simulink model "VelocityControlPI"  (R2022a)
settings: Solver=VariableStepAuto  StartTime=0.0  StopTime=inf  RelTol=1e-3
undefined symbols (not defined in the file): a, b, k1, k2
libraries: arduinolib x4, arduinosensorlib x2
settings Model: Creator=LabPC  LastModifiedBy=LabPC

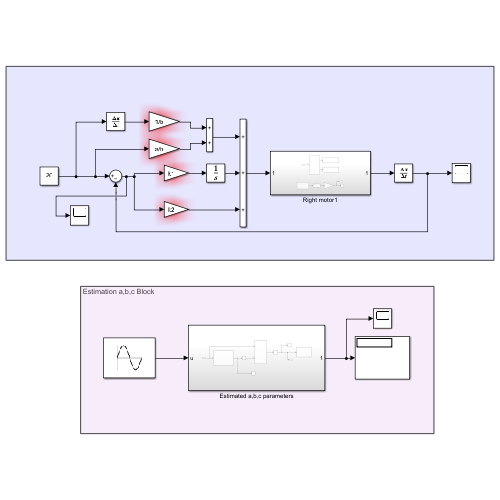
[thumbnail: Simulink's stored preview of the top-level diagram]
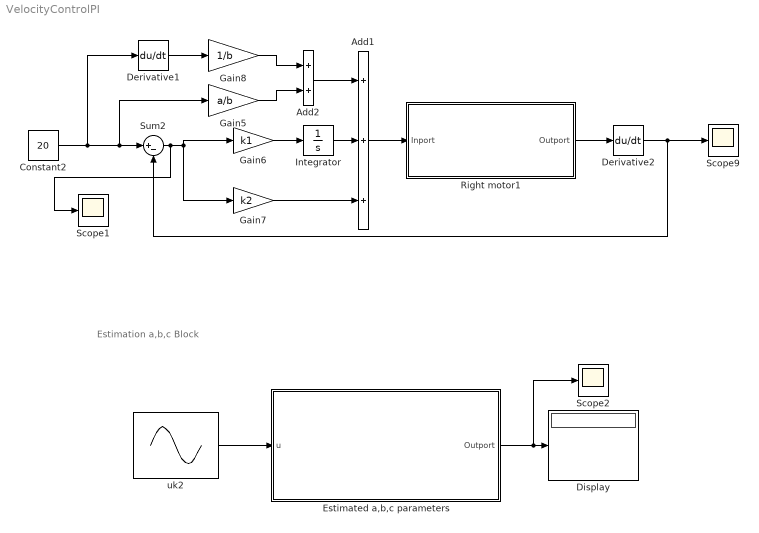
== system VelocityControlPI ==
  note: Estimation a,b,c Block
  Add1 : Sum  Inputs=+++
  Add2 : Sum
  Constant2 : Constant  Value=20
  Derivative1 : Derivative
  Derivative2 : Derivative
  Display : Display
  Estimated a,b,c parameters : Subsystem
  Gain5 : Gain  Gain=a/b
  Gain6 : Gain  Gain=k1
  Gain7 : Gain  Gain=k2
  Gain8 : Gain  Gain=1/b
  Integrator : Integrator
  Right motor1 : Subsystem
  Scope1 : Scope
  Scope2 : Scope
  Scope9 : Scope
  Sum2 : Sum  Inputs=|+-
  uk2 : Sin  Amplitude=14  Frequency=2*pi*1  SampleTime=0
  wires:
  Gain8/1 -> Add2/1
  Gain6/1 -> Integrator/1
  Right motor1/1(Outport) -> Derivative2/1
  Sum2/1 -> Scope1/1, Gain6/1, Gain7/1
  Derivative1/1 -> Gain8/1
  Integrator/1 -> Add1/2
  Add1/1 -> Right motor1/1(Inport)
  Add2/1 -> Add1/1
  Derivative2/1 -> Scope9/1, Sum2/2
  Gain7/1 -> Add1/3
  Gain5/1 -> Add2/2
  Constant2/1 -> Gain5/1, Sum2/1, Derivative1/1
  uk2/1 -> Estimated a,b,c parameters/1(u)
  Estimated a,b,c parameters/1(Outport) -> Scope2/1, Display/1

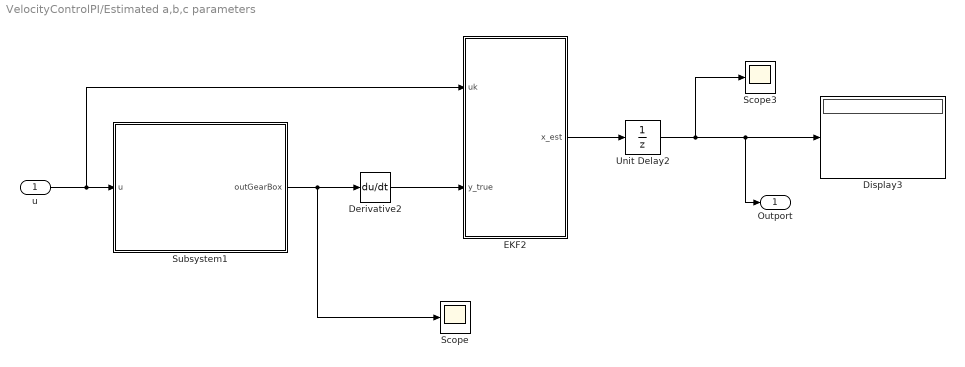
== system VelocityControlPI/Estimated a,b,c parameters ==
  u : Inport
  Derivative2 : Derivative
  Display3 : Display
  EKF2 : MATLAB Function  TreatAsAtomicUnit=on
  Scope : Scope
  Scope3 : Scope
  Subsystem1 : Subsystem
  Unit Delay2 : UnitDelay  InitialCondition=[0;0;0;0]  SampleTime=-1  HasFrameUpgradeWarning=on
  Outport : Outport
  wires:
  Derivative2/1 -> EKF2/2(y_true)
  Unit Delay2/1 -> Outport/1, Display3/1, Scope3/1
  EKF2/1(x_est) -> Unit Delay2/1
  Subsystem1/1(outGearBox) -> Scope/1, Derivative2/1
  u/1 -> EKF2/1(uk), Subsystem1/1(u)

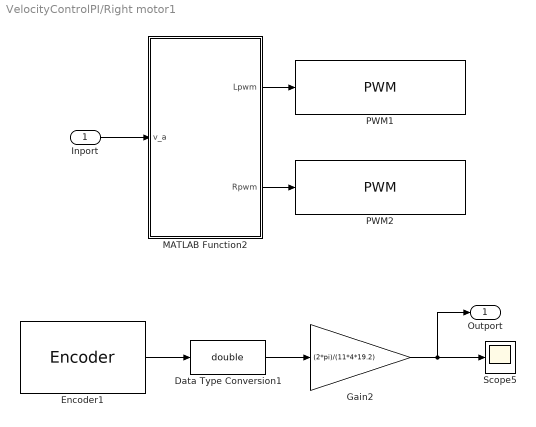
== system VelocityControlPI/Right motor1 ==
  Inport : Inport
  Data Type Conversion1 : DataTypeConversion  OutDataTypeStr=double  SaturateOnIntegerOverflow=off  RndMeth=Floor
  Encoder1 : arduinosensorlib/Encoder  InputA=2  InputB=3  Mode=No reset  SampleTime=-1
      settings: SourceProductBaseCode=ARDUINO
  Gain2 : Gain  Gain=(2*pi)/(11*4*19.2)
  MATLAB Function2 : MATLAB Function  TreatAsAtomicUnit=on
  PWM1 : arduinolib/PWM  pinNumber=8  frequencyType=Default  desiredFrequency=490.2  achievableFrequency=490.2
  PWM2 : arduinolib/PWM  pinNumber=9  frequencyType=Default  desiredFrequency=490.2  achievableFrequency=490.2
  Scope5 : Scope
  Outport : Outport
  wires:
  Gain2/1 -> Scope5/1, Outport/1
  Data Type Conversion1/1 -> Gain2/1
  Encoder1/1 -> Data Type Conversion1/1
  Inport/1 -> MATLAB Function2/1(v_a)
  MATLAB Function2/1(Lpwm) -> PWM1/1
  MATLAB Function2/2(Rpwm) -> PWM2/1

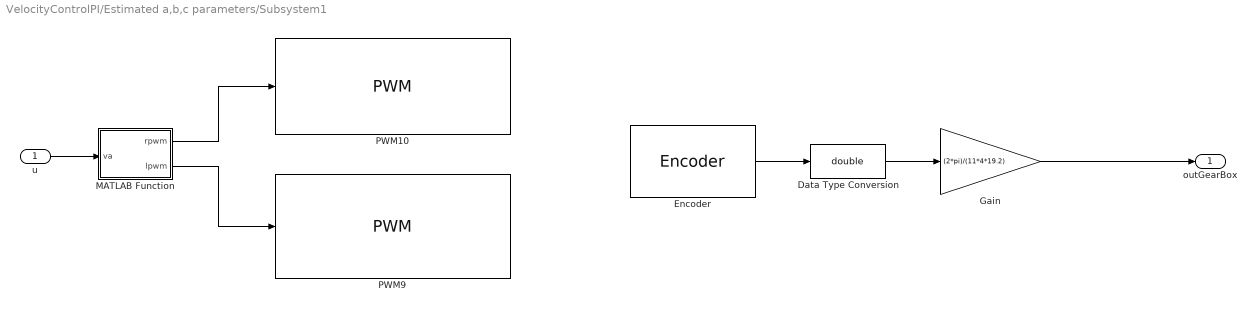
== system VelocityControlPI/Estimated a,b,c parameters/Subsystem1 ==
  u : Inport
  Data Type Conversion : DataTypeConversion  OutDataTypeStr=double  SaturateOnIntegerOverflow=off  RndMeth=Floor
  Encoder : arduinosensorlib/Encoder  InputA=2  InputB=3  Mode=No reset  SampleTime=-1
      settings: SourceProductBaseCode=ARDUINO
  Gain : Gain  Gain=(2*pi)/(11*4*19.2)
  MATLAB Function : MATLAB Function  TreatAsAtomicUnit=on
  PWM10 : arduinolib/PWM  pinNumber=8  frequencyType=Default  desiredFrequency=490.2  achievableFrequency=490.2
  PWM9 : arduinolib/PWM  pinNumber=9  frequencyType=Default  desiredFrequency=490.2  achievableFrequency=490.2
  outGearBox : Outport
  wires:
  Gain/1 -> outGearBox/1
  u/1 -> MATLAB Function/1(va)
  MATLAB Function/1(rpwm) -> PWM10/1
  MATLAB Function/2(lpwm) -> PWM9/1
  Encoder/1 -> Data Type Conversion/1
  Data Type Conversion/1 -> Gain/1

== matlab function VelocityControlPI/Estimated a,b,c parameters/Subsystem1/MATLAB Function ==
  data: va input; rpwm output; lpwm output
function [rpwm,lpwm] = fcn(va)

pwm = (va/24)*254;

if pwm > 0
    rpwm = pwm;
    lpwm = 0;
elseif pwm<0
    rpwm = 0;
    lpwm = abs(pwm);
else
    rpwm = 0;
    lpwm = 0;
end

== matlab function VelocityControlPI/Right motor1/MATLAB Function2 ==
  data: v_a input; Lpwm output; Rpwm output
function [Lpwm,Rpwm] = fcn(v_a)

vmax = 22.9;
pwm_cal = v_a*254/vmax;

if pwm_cal > 0
    Lpwm = 0;
    Rpwm = pwm_cal;
elseif pwm_cal < 0
    Lpwm = abs(pwm_cal);
    Rpwm = 0;
else
    Lpwm = 0;
    Rpwm = 0;
end

== matlab function VelocityControlPI/Estimated a,b,c parameters/EKF2 ==
  settings: updateMethod=DISCRETE
  data: uk input; y_true input; x_est output
function x_est = fcn(uk,y_true)
Ts=0.01;
persistent x_est_p P Qd_est R_est Qc_est;
if isempty(x_est_p)
          
          x_est_p=[2;13;25;1];
          P=2*eye(4);
         Qc_est=1e-5*diag([10,25,25,1]);
          Qd_est=Qc_est*Ts;
          R_est=0.02;
end
c=[1 0 0 0];D=0;Ck=c;Dk=D;
%Comput Kalman Gain and update predicted value
Wk=P*Ck'/(Ck*P*Ck'+R_est);
y_est=Ck*x_est_p+Dk*uk;
x=x_est_p+Wk.*(y_true-y_est);
%Compute prediction at next time step
x_est=x+Ts*[-x(2)*x(1)+uk*x(3)-x(4)*sign(x(1));0;0;0];
%Update error covariance matrices
P=P-Wk*Ck*P;
%Define Ak
Ak=eye(4)+Ts*[-x(2) -x(1) uk -sign(x(1));0 0 0 0;0 0 0 0;0 0 0 0];
P=Ak*P*Ak'+Qd_est;
x_est_p=x_est;
